simulink model "ball_beam_simulink"  (R2014b)
settings: Solver=ode45  StartTime=0.0  StopTime=10.0  RelTol=1e-3
values from neighbouring files (symbols this model uses):
  Bm = 0.01    [ball.m]    (also in ball_and_beam.m; tham_so.m)
  Jm = 0.000052    (= 5.2e-05)    [ball.m]    (also in ball_and_beam.m; tham_so.m)
  Ke = 0.235    [ball.m]    (also in ball_and_beam.m; tham_so.m)
  Kt = 0.235    [ball.m]    (also in ball_and_beam.m; tham_so.m)
  La = 0.23    [ball.m]    (also in ball_and_beam.m; tham_so.m)
  Ra = 2    [ball.m]    (also in ball_and_beam.m; tham_so.m)
settings Model: Creator=Admin  LastModifiedBy=Admin

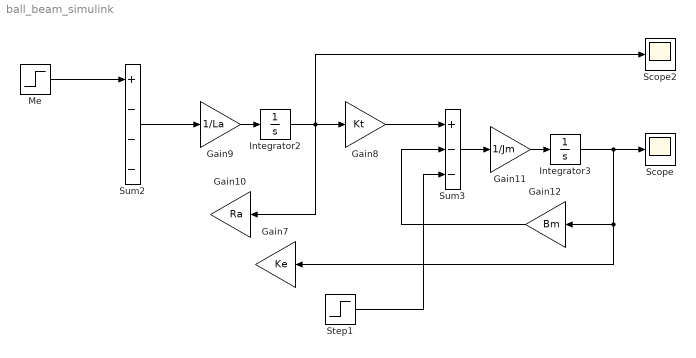
== system ball_beam_simulink ==
  Gain10 : Gain  Gain=Ra
  Gain11 : Gain  Gain=1/Jm
  Gain12 : Gain  Gain=Bm
  Gain7 : Gain  Gain=Ke
  Gain8 : Gain  Gain=Kt
  Gain9 : Gain  Gain=1/La
  Integrator2 : Integrator
  Integrator3 : Integrator
  Me : Step  Time=0  SampleTime=0
  Scope : Scope
      settings: YMin=0  YMax=10
  Scope2 : Scope
      settings: YMin=0  YMax=10  SaveName=ScopeData2
  Step1 : Step  Time=0  After=0  SampleTime=0
  Sum2 : Sum  Inputs=+---
  Sum3 : Sum  Inputs=+--
  wires:
  Gain9/1 -> Integrator2/1
  Gain8/1 -> Sum3/1
  Sum3/1 -> Gain11/1
  Gain11/1 -> Integrator3/1
  Gain12/1 -> Sum3/2
  Me/1 -> Sum2/1
  Step1/1 -> Sum3/3
  Integrator3/1 -> Gain7/1, Gain12/1, Scope/1
  Integrator2/1 -> Scope2/1, Gain10/1, Gain8/1
  Sum2/1 -> Gain9/1
